simulink model "pendSimPID"  (R2024a)
settings: Solver=FixedStepAuto  StartTime=0.0  StopTime=15  FixedStep=0.001  MaxStep=0.005  RelTol=1e-3
libraries: simulink x1
settings Model: Creator=mattf  LastModifiedBy=ariellevy

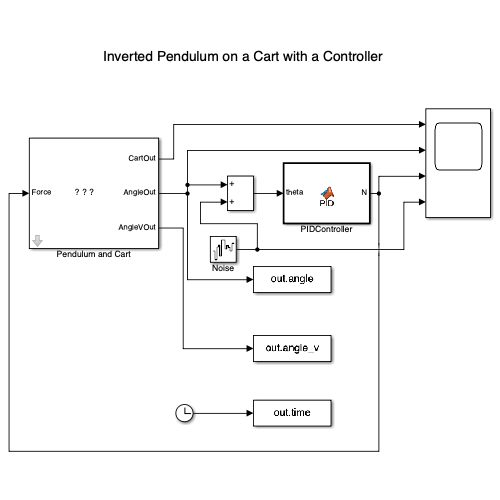
[thumbnail: Simulink's stored preview of the top-level diagram]
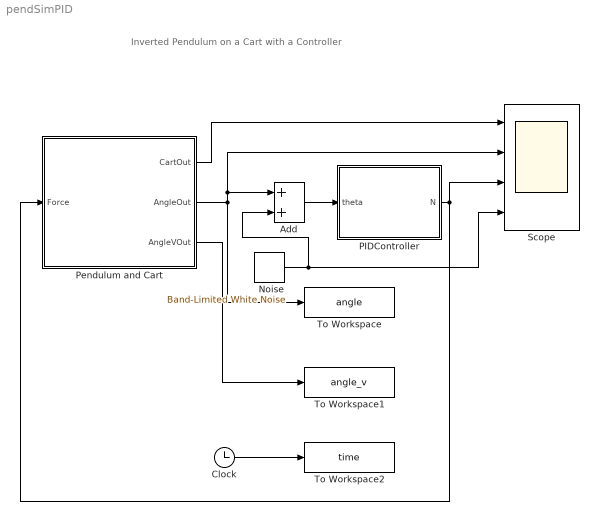
== system pendSimPID ==
  note: Inverted Pendulum on a Cart with a Controller
  Add : Sum
  Clock : Clock
  Noise : simulink/Sources/Band-Limited White Noise  Cov=[0.00001]  Ts=0.001  seed=[23341]
  PIDController : MATLAB Function  TreatAsAtomicUnit=on  SystemSampleTime=0.001
  Pendulum and Cart : Subsystem  SystemSampleTime=0.001  mask{Mcart=0.5, m=0.2, l=0.3/2, g=9.8, init=pi/6}
      mask prompts: Mcart "Cart Mass (kg):"; m "Pend Mass (kg):"; l "COM Distance (m):"; g "Acc due to Gravity (g):"; init "Initial Angle (rad):"
      mask Display: image('pen img.png');
  Scope : Scope  NumInputPorts=4
  To Workspace : ToWorkspace  VariableName=angle  SampleTime=0.005
  To Workspace1 : ToWorkspace  VariableName=angle_v  SampleTime=0.005
  To Workspace2 : ToWorkspace  VariableName=time  SampleTime=0.005
  wires:
  Clock/1 -> To Workspace2/1
  Pendulum and Cart/3(AngleVOut) -> To Workspace1/1
  Pendulum and Cart/1(CartOut) -> Scope/1
  Pendulum and Cart/2(AngleOut) -> Add/1, Scope/2, To Workspace/1
  PIDController/1(N) -> Pendulum and Cart/1(Force), Scope/3
  Add/1 -> PIDController/1(theta)
  Noise/1 -> Scope/4, Add/2

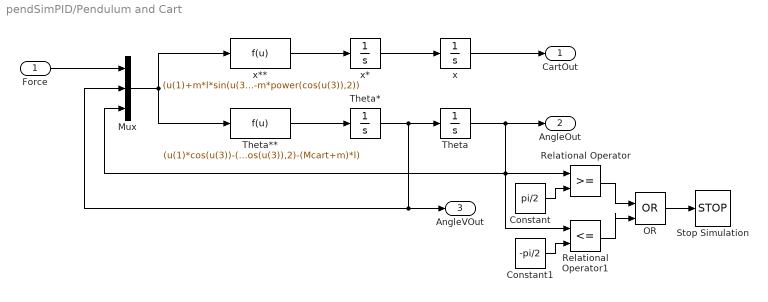
== system pendSimPID/Pendulum and Cart ==
  Force : Inport
  Constant : Constant  Value=pi/2
  Constant1 : Constant  Value=-pi/2
  Mux : Mux  Inputs=3
  OR : Logic  Operator=OR  IconShape=distinctive  AllPortsSameDT=off  OutDataTypeStr=boolean
  Relational Operator : RelationalOperator  OutDataTypeStr=boolean  RndMeth=Simplest  InputSameDT=off
  Relational Operator1 : RelationalOperator  Operator=<=  OutDataTypeStr=boolean  RndMeth=Simplest  InputSameDT=off
  Stop Simulation : Stop
  Theta : Integrator  InitialCondition=init
  Theta* : Integrator
  Theta** : Fcn  Expr=(u(1)*cos(u(3))-(Mcart+m)*g*sin(u(3))+m*l*cos(u(3))*sin(u(3))*power(u(2),2))/(m*l*power(cos(u(3)),2)-(Mcart+m)*l)
  x : Integrator
  x* : Integrator
  x** : Fcn  Expr=(u(1)+m*l*sin(u(3))*power(u(2),2)-m*g*cos(u(3))*sin(u(3)))/(Mcart+m-m*power(cos(u(3)),2))
  CartOut : Outport
  AngleOut : Outport  Port=2
  AngleVOut : Outport  Port=3
  wires:
  Mux/1 -> x**/1, Theta**/1
  x*/1 -> x/1
  x/1 -> CartOut/1
  Force/1 -> Mux/1
  Theta**/1 -> Theta*/1
  x**/1 -> x*/1
  Theta*/1 -> Mux/2, AngleVOut/1, Theta/1
  Theta/1 -> AngleOut/1, Relational Operator1/1, Relational Operator/1, Mux/3
  Constant/1 -> Relational Operator/2
  Constant1/1 -> Relational Operator1/2
  OR/1 -> Stop Simulation/1
  Relational Operator1/1 -> OR/2
  Relational Operator/1 -> OR/1

== matlab function pendSimPID/PIDController ==
  settings: updateMethod=DISCRETE
  data: N output; theta input
function N = PID(theta)

    % call extrinsic python function
    coder.extrinsic('py.PIDController.controller_call');

    % Call Python function and return result
    N = coder.nullcopy(zeros(1,1)); % no clue why, but this is need.
    N = double(py.PIDController.controller_call(0, theta));
    end
